simulink model "ex1desen"  (R2025b)
settings: Solver=VariableStepAuto  StartTime=0.0  StopTime=10.0  RelTol=1e-3
libraries: simulink x1

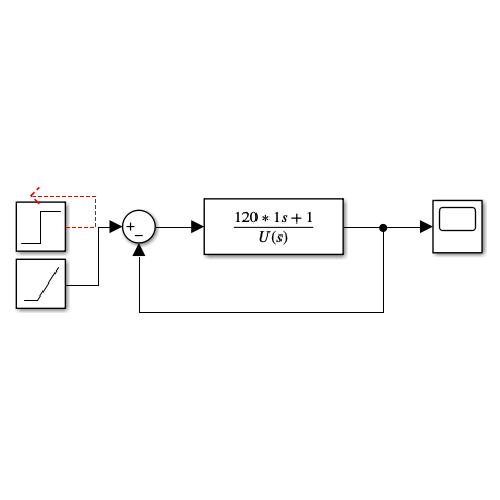
[thumbnail: Simulink's stored preview of the top-level diagram]
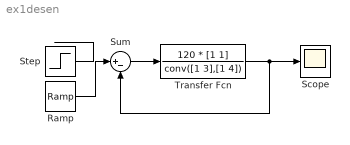
== system ex1desen ==
  Ramp : simulink/Sources/Ramp  slope=1  start=0  InitialOutput=0
  Scope : Scope
      settings: ActiveDisplayYMinimum=-1.1406707728582886  ActiveDisplayYMaximum=10.2660369557246
  Step : Step  SampleTime=0
  Sum : Sum  Inputs=|+-
  Transfer Fcn : TransferFcn  Numerator=120 * [1 1]  Denominator=conv([1 3],[1 4])
  wires:
  Sum/1 -> Transfer Fcn/1
  Step/1 -> ?
  Transfer Fcn/1 -> Scope/1, Sum/2
  Ramp/1 -> Sum/1
